simulink model "SIMULACION_HUMMINGBIRD_ACELERACION"  (R2024b)
settings: Solver=FixedStepAuto  StartTime=0.0  StopTime=10  FixedStep=1e-3  RelTol=1e-3
settings Model: Creator=Raul Robles  LastModifiedBy=Raul Robles

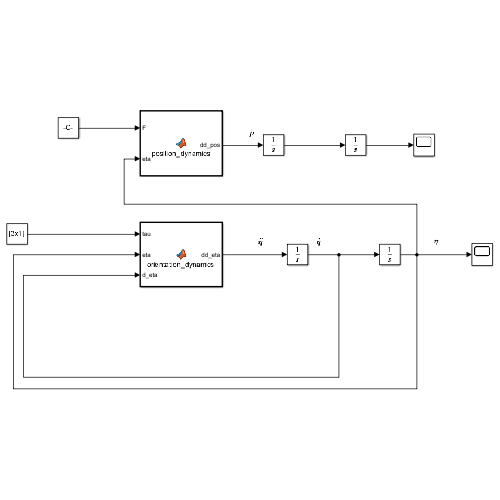
[thumbnail: Simulink's stored preview of the top-level diagram]
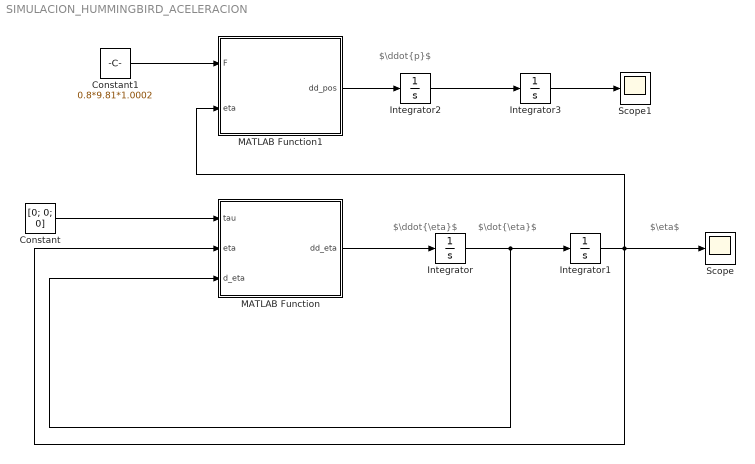
== system SIMULACION_HUMMINGBIRD_ACELERACION ==
  note: $\ddot{p}$
  note: $\dot{\eta}$
  note: $\eta$
  note: $\ddot{\eta}$
  Constant : Constant  Value=[0; 0; 0]
  Constant1 : Constant  Value=0.8*9.81*1.0002
  Integrator{,1..3} (4 alike) : Integrator  InitialCondition=[0; 0; 0]
  MATLAB Function : MATLAB Function  TreatAsAtomicUnit=on
  MATLAB Function1 : MATLAB Function  TreatAsAtomicUnit=on
  Scope : Scope
  Scope1 : Scope
  wires:
  MATLAB Function/1(dd_eta) -> Integrator/1
  Constant/1 -> MATLAB Function/1(tau)
  Integrator1/1 -> MATLAB Function1/2(eta), MATLAB Function/2(eta), Scope/1
  Integrator/1 -> MATLAB Function/3(d_eta), Integrator1/1
  Constant1/1 -> MATLAB Function1/1(F)
  MATLAB Function1/1(dd_pos) -> Integrator2/1
  Integrator2/1 -> Integrator3/1
  Integrator3/1 -> Scope1/1

== matlab function SIMULACION_HUMMINGBIRD_ACELERACION/MATLAB Function ==
  data: tau input; dd_eta output; eta input; d_eta input
function dd_eta = orientation_dynamics(tau, eta, d_eta)
    
    % Matriz de inercia (momento de inercia)
    Ixx = 0.00273;
    Iyy = 0.00273;
    Izz = 0.00541;
    I = diag([Ixx, Iyy, Izz]);

    % Matriz de transformación PHI
    PHI_11 = 1;
    PHI_12 = sin(eta(1))*tan(eta(2));
    PHI_13 = cos(eta(1))*tan(eta(2));
    PHI_21 = 0;
    PHI_22 = cos(eta(1));
    PHI_23 = -sin(eta(1));
    PHI_31 = 0;
    PHI_32 = sin(eta(1))/cos(eta(2));
    PHI_33 = cos(eta(1))/cos(eta(2));

    PHI = [
        PHI_11, PHI_12, PHI_13;
        PHI_21, PHI_22, PHI_23;
        PHI_31, PHI_32, PHI_33
    ];
    
    % Derivada de la matriz PHI
    PHI_D_11 = 0;
    PHI_D_12 = d_eta(1)*cos(eta(1))*tan(eta(2)) + d_eta(2)*(sin(eta(1))/(cos(eta(2))^2));
    PHI_D_13 = d_eta(2)*(cos(eta(1))/(cos(eta(2))^2)) - d_eta(1)*sin(eta(1))*tan(eta(2));
    PHI_D_21 = 0;
    PHI_D_22 = -d_eta(1)*sin(eta(1));
    PHI_D_23 = -d_eta(1)*cos(eta(1));
    PHI_D_31 = 0;
    PHI_D_32 = (cos(eta(1))*cos(eta(2))*d_eta(1) + sin(eta(1))*sin(eta(2))*d_eta(2))/(cos(eta(2))^2);
    PHI_D_33 = (cos(eta(1))*sin(eta(2))*d_eta(2) - sin(eta(1))*cos(eta(2))*d_eta(1))/(cos(eta(2))^2);
    
    PHI_D = [
        PHI_D_11, PHI_D_12, PHI_D_13;
        PHI_D_21, PHI_D_22, PHI_D_23;
        PHI_D_31, PHI_D_32, PHI_D_33
    ];
    
   
    PHI_inv = inv(PHI); %%Inversa de la matriz PHI
    M = (PHI_inv') * I * PHI_inv; %%% Matriz M
    M_1 = inv(M); %%Inversa de la matriz M
    
    % Matriz S
    S = [0 -1 1; 1 0 -1; -1 1 0];
    
    % Matriz Coriolis
    C = (PHI_inv') * (S * (I * (PHI_inv)) - I * (PHI_inv) * PHI_D) * PHI_inv;
    
    fn = (PHI_inv') * tau; 

    % Cálculo de la aceleración angular
    dd_eta = (M_1) * (-C * d_eta + fn);
end

== matlab function SIMULACION_HUMMINGBIRD_ACELERACION/MATLAB Function1 ==
  data: F input; dd_pos output; eta input
function dd_pos = position_dynamics(F, eta)
    
%%% Masa del quad
m = 0.8; %%%[kg]

%%% Vector de gravedad
g = 9.81;
gz = [0; 0; g];

%%% Matriz de rotacion

R_11 = cos(eta(2))*cos(eta(3));
R_12 = sin(eta(1))*sin(eta(2))*cos(eta(3)) - cos(eta(1))*sin(eta(3));
R_13 = cos(eta(1))*sin(eta(2))*cos(eta(3)) + sin(eta(1))*sin(eta(3));
R_21 = cos(eta(2))*sin(eta(3));
R_22 = sin(eta(1))*sin(eta(2))*sin(eta(3)) + cos(eta(1))*cos(eta(3));
R_23 = cos(eta(1))*sin(eta(2))*sin(eta(3)) - sin(eta(1))*cos(eta(3));
R_31 = -sin(eta(2));
R_32 = sin(eta(1))*cos(eta(2));
R_33 = cos(eta(1))*cos(eta(2));

R = [R_11 R_12 R_13; R_21 R_22 R_23; R_31 R_32 R_33];

%%%% Vector r3

r3 = R*[0; 0; 1];

%%% Vector fp (fuerza en el marco de referencia inercial)

fp = r3*F;
% Dinámica de la posición
    dd_pos = (1/m)*fp - gz;
end
